simulink model "bfsk"  (R2016a)
settings: Solver=VariableStepAuto  StartTime=0.0  StopTime=1000  RelTol=1e-3
libraries: dsparch4 x4, commchan3 x1, commrandsrc3 x1, commsink2 x1
settings Model: Creator=hp  LastModifiedBy=hp

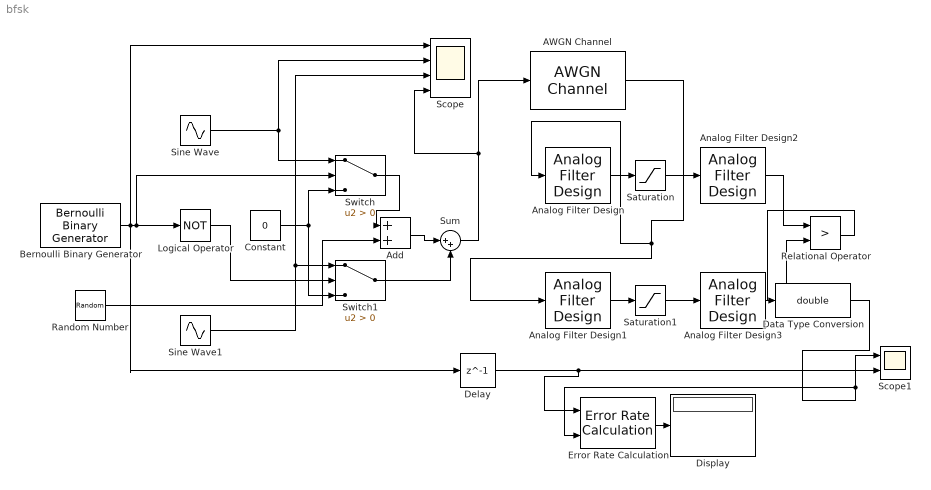
== system bfsk ==
  AWGN Channel : commchan3/AWGN Channel  InputProcessing=Columns as channels (frame based)  seed=67  noiseMode=Variance from mask  EbNodB=30  EsNodB=10  SNRdB=10  bitsPerSym=1  Ps=1  Tsym=1  variance=0.2
  Add : Sum
  Analog Filter Design : dsparch4/Analog Filter Design  method=Butterworth  filttype=Bandpass  N=8  Wlo=80  Whi=120  Rp=2  Rs=40
  Analog Filter Design1 : dsparch4/Analog Filter Design  method=Butterworth  filttype=Bandpass  N=8  Wlo=10  Whi=30  Rp=2  Rs=40
  Analog Filter Design2 : dsparch4/Analog Filter Design  method=Butterworth  filttype=Lowpass  N=8  Wlo=10  Whi=80  Rp=2  Rs=40
  Analog Filter Design3 : dsparch4/Analog Filter Design  method=Butterworth  filttype=Lowpass  N=8  Wlo=10  Whi=80  Rp=2  Rs=40
  Bernoulli Binary Generator : commrandsrc3/Bernoulli Binary Generator  ProbabilityOfZero=0.5  SeedSource=Parameter  Seed=61  SampleTime=1  SamplesPerFrame=1  OutputDataType=double  SimulateUsing=Interpreted execution
  Constant : Constant  Value=0
  Data Type Conversion : DataTypeConversion  OutDataTypeStr=double
  Delay : Delay  DelayLength=1  InitialCondition=0
  Display : Display
  Error Rate Calculation : commsink2/Error Rate Calculation  N=0  st_delay=0  cp_mode=Entire frame  subframe=[]  PMode=Port  WsName=ErrorVec  RsMode2=off  stop=off  numErr=100  maxBits=1e6
  Logical Operator : Logic  Operator=NOT  Inputs=1  AllPortsSameDT=off
  Random Number : RandomNumber  Seed=41  SampleTime=1
  Relational Operator : RelationalOperator  Operator=>  OutDataTypeStr=boolean
  Saturation : Saturate  UpperLimit=inf  LowerLimit=0
  Saturation1 : Saturate  UpperLimit=inf  LowerLimit=0
  Scope : Scope  NumInputPorts=4
  Scope1 : Scope  NumInputPorts=2
  Sine Wave : Sin  Frequency=100  SampleTime=0
  Sine Wave1 : Sin  Frequency=20  SampleTime=0
  Sum : Sum  Inputs=|++
  Switch : Switch  Criteria=u2 > Threshold
  Switch1 : Switch  Criteria=u2 > Threshold
  wires:
  Sine Wave/1 -> Scope/2, Switch/1
  Constant/1 -> Switch1/3, Switch/3
  Switch1/1 -> Sum/2
  Sine Wave1/1 -> Scope/3, Switch1/1
  Logical Operator/1 -> Switch1/2
  Sum/1 -> Scope/4, AWGN Channel/1
  Analog Filter Design/1 -> Saturation/1
  Analog Filter Design1/1 -> Saturation1/1
  Saturation/1 -> Analog Filter Design2/1
  Saturation1/1 -> Analog Filter Design3/1
  Analog Filter Design2/1 -> Relational Operator/1
  Analog Filter Design3/1 -> Relational Operator/2
  Switch/1 -> Add/1
  Random Number/1 -> Add/2
  Add/1 -> Sum/1
  AWGN Channel/1 -> Analog Filter Design1/1, Analog Filter Design/1
  Error Rate Calculation/1 -> Display/1
  Bernoulli Binary Generator/1 -> Delay/1, Scope/1, Switch/2, Logical Operator/1
  Relational Operator/1 -> Data Type Conversion/1
  Delay/1 -> Error Rate Calculation/1, Scope1/2
  Data Type Conversion/1 -> Scope1/1, Error Rate Calculation/2
